simulink model "cyborg"  (R2018b)
settings: Solver=ode4  StartTime=0.0  StopTime=inf  FixedStep=0.01  RelTol=1e-3
undefined symbols (not defined in the file): f
libraries: instrumentlib x2, dsparch4 x1, dspstat3 x1
settings Model: Creator=oscar  LastModifiedBy=oscar

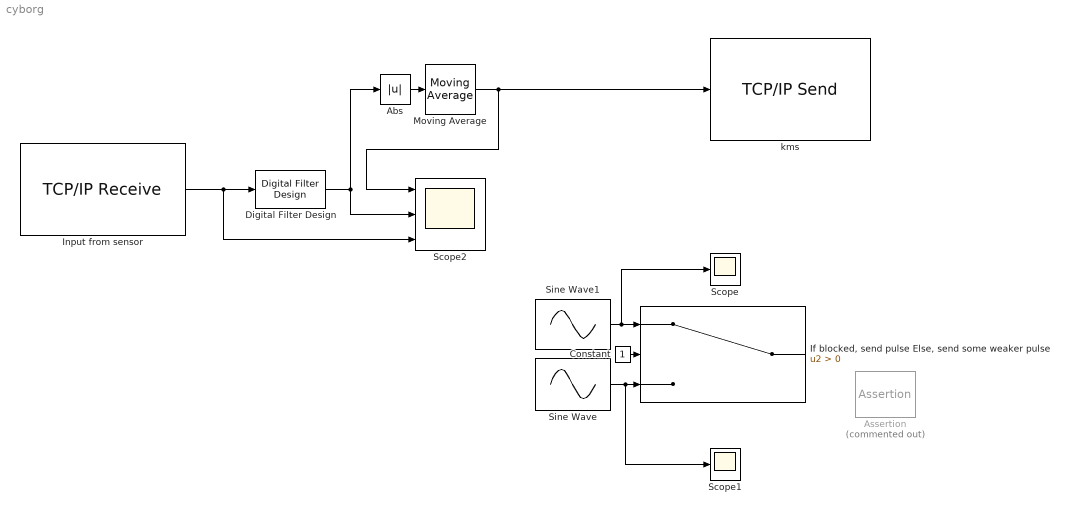
== system cyborg ==
  Abs : Abs
  Assertion : Assertion  Commented=on
  Constant : Constant
  Digital Filter Design : dsparch4/Digital Filter Design  mwdsp_browser_bugfix_var=off
  "If blocked, send pulse Else, send some weaker pulse" : Switch  Criteria=u2 > Threshold
  Input from sensor : instrumentlib/TCP//IP Receive  Host=10.24.35.227  Port=8080  DataSize="[100    1]"  EnableBlockingMode=on  Timeout=10  SampleTime=-1  DataType=single  ByteOrder=LittleEndian  ASCIIFormatting=%f,  Terminator=LF
      settings: SourceProductName=Instrument Control Toolbox
  Moving Average : dspstat3/Moving Average  Method=Sliding window  ForgettingFactorPort=off  SpecifyWindowLength=on  WindowLength=10000  ForgettingFactor=0.9  SimulateUsing=Interpreted execution
  Scope : Scope
  Scope1 : Scope
  Scope2 : Scope  NumInputPorts=3
  Sine Wave : Sin  Frequency=10  SampleTime=0
  Sine Wave1 : Sin  Frequency=pi  SampleTime=0
  kms : instrumentlib/TCP//IP Send  Host=10.24.35.227  Port=8081  EnableBlockingMode=on  Timeout=10  ByteOrder=BigEndian  TransferDelay=on
      settings: SourceProductName=Instrument Control Toolbox
  wires:
  Sine Wave/1 -> Scope1/1, "If blocked, send pulse Else, send some weaker pulse"/3
  Sine Wave1/1 -> Scope/1, "If blocked, send pulse Else, send some weaker pulse"/1
  Constant/1 -> "If blocked, send pulse Else, send some weaker pulse"/2
  Input from sensor/1 -> Scope2/3, Digital Filter Design/1
  Digital Filter Design/1 -> Scope2/2, Abs/1
  Abs/1 -> Moving Average/1
  Moving Average/1 -> kms/1, Scope2/1
